simulink model "raibert_controller_running"  (R2018b)
settings: Solver=FixedStepDiscrete  StartTime=0.0  StopTime=inf  FixedStep=sample_time  RelTol=1e-3
InitFcn:
  | warning off all
undefined symbols (not defined in the file or in its folder): ctrl, Discrete, initial_dx_estimate, initial_dy_estimate, initial_dz_estimate, initial_z_estimate, sample_time, Time
libraries: simulink x27, ctrlSharedLib x7
(part 4 of 4)

== matlab function raibert_controller_running/Behavior/Primary-Secondary Routing Inputs ==
  data: right_is_primary input size=1; leg_angle_primary output size=2; leg_angle_right input size=2; leg_length_right input size=2; leg_width_right input size=2; leg_roll_right input size=2; back_load_right input size=2; back_motor_right input size=2; front_load_right input size=2; front_motor_right input size=2; lateral_right input size=2; axial_force_right input; grf_xz_right input; foot2com_x_right input; foot2com_z_right input; x_state_right input; leg_angle_left input size=2; leg_length_left input size=2; leg_width_left input size=2; leg_roll_left input size=2; back_load_left input size=2; back_motor_left input size=2; front_load_left input size=2; front_motor_left input size=2; lateral_left input size=2; leg_length_primary output size=2; leg_width_primary output size=2; leg_roll_primary output size=2; back_load_primary output size=2; back_motor_primary output size=2; front_load_primary output size=2; front_motor_primary output size=2; lateral_primary output size=2; axial_force_primary output; grf_xz_primary output; foot2com_x_primary output; foot2com_z_primary output; x_state_primary output; leg_angle_secondary output size=2; leg_length_secondary output size=2; leg_width_secondary output size=2; leg_roll_secondary output size=2; back_load_secondary output size=2; back_motor_secondary output size=2; front_load_secondary output size=2; front_motor_secondary output size=2; lateral_secondary output size=2; axial_force_left input; grf_xz_left input; foot2com_x_left input; foot2com_z_left input; axial_force_secondary output; grf_xz_secondary output; foot2com_x_secondary output; foot2com_z_secondary output; x_state_secondary output; x_state_left input
% Switch between "primary" and "secondary" leg variables
function [leg_angle_primary, ...
          leg_length_primary, ...
          leg_width_primary, ...
          leg_roll_primary, ...
          back_load_primary, ...
          back_motor_primary, ...
          front_load_primary, ...
          front_motor_primary, ...
          lateral_primary, ...
          axial_force_primary, ...
          grf_xz_primary, ...
          foot2com_x_primary, ...
          foot2com_z_primary, ...
          x_state_primary, ...
          leg_angle_secondary, ...
          leg_length_secondary, ...
          leg_width_secondary, ...
          leg_roll_secondary, ...
          back_load_secondary, ...
          back_motor_secondary, ...
          front_load_secondary, ...
          front_motor_secondary, ...
          lateral_secondary, ...
          axial_force_secondary, ...
          grf_xz_secondary, ...
          foot2com_x_secondary, ...
          foot2com_z_secondary, ...
          x_state_secondary] ...
          = SignalSwitch(...
          right_is_primary, ...
          leg_angle_right, ...
          leg_length_right, ...
          leg_width_right, ...
          leg_roll_right, ...
          back_load_right, ...
          back_motor_right, ...
          front_load_right, ...
          front_motor_right, ...
          lateral_right, ...
          axial_force_right, ...
          grf_xz_right, ...
          foot2com_x_right, ...
          foot2com_z_right, ...
          x_state_right, ...
          leg_angle_left, ...
          leg_length_left, ...
          leg_width_left, ...
          leg_roll_left, ...
          back_load_left, ...
          back_motor_left, ...
          front_load_left, ...
          front_motor_left, ...
          lateral_left, ...
          axial_force_left, ...
          grf_xz_left, ...
          foot2com_x_left, ...
          foot2com_z_left, ...
          x_state_left)

if right_is_primary % right leg is primary
  leg_angle_primary = leg_angle_right;
  leg_length_primary = leg_length_right;
  leg_width_primary = leg_width_right;
  leg_roll_primary = leg_roll_right;
  back_load_primary = back_load_right;
  back_motor_primary = back_motor_right;
  front_load_primary = front_load_right;
  front_motor_primary = front_motor_right;
  lateral_primary = lateral_right;
  axial_force_primary = axial_force_right;
  grf_xz_primary = grf_xz_right;
  foot2com_x_primary = foot2com_x_right;
  foot2com_z_primary = foot2com_z_right;
  x_state_primary = x_state_right;
  leg_angle_secondary = leg_angle_left;
  leg_length_secondary = leg_length_left;
  leg_width_secondary = leg_width_left;
  leg_roll_secondary = leg_roll_left;
  back_load_secondary = back_load_left;
  back_motor_secondary = back_motor_left;
  front_load_secondary = front_load_left;
  front_motor_secondary = front_motor_left;
  lateral_secondary = lateral_left;
  axial_force_secondary = axial_force_left;
  grf_xz_secondary = grf_xz_left;
  foot2com_x_secondary = foot2com_x_left;
  foot2com_z_secondary = foot2com_z_left;
  x_state_secondary = x_state_left;
else % left leg is primary
  leg_angle_primary = leg_angle_left;
  leg_length_primary = leg_length_left;
  leg_width_primary = leg_width_left;
  leg_roll_primary = leg_roll_left;
  back_load_primary = back_load_left;
  back_motor_primary = back_motor_left;
  front_load_primary = front_load_left;
  front_motor_primary = front_motor_left;
  lateral_primary = lateral_left;
  axial_force_primary = axial_force_left;
  grf_xz_primary = grf_xz_left;
  foot2com_x_primary = foot2com_x_left;
  foot2com_z_primary = foot2com_z_left;
  x_state_primary = x_state_left;
  leg_angle_secondary = leg_angle_right;
  leg_length_secondary = leg_length_right;
  leg_width_secondary = leg_width_right;
  leg_roll_secondary = leg_roll_right;
  back_load_secondary = back_load_right;
  back_motor_secondary = back_motor_right;
  front_load_secondary = front_load_right;
  front_motor_secondary = front_motor_right;
  lateral_secondary = lateral_right;
  axial_force_secondary = axial_force_right;
  grf_xz_secondary = grf_xz_right;
  foot2com_x_secondary = foot2com_x_right;
  foot2com_z_secondary = foot2com_z_right;
  x_state_secondary = x_state_right;
end

== matlab function raibert_controller_running/Behavior/Filtering/Kalman Filtering/Measurement Noise Covariance Matricies ==
  data: R_no_position output; R_transverse_right output; R_transverse_left output; vertical_GRF_L input; vertical_GRF_R input; sample_time parameter; ctrl parameter; R_vertical output
function [R_no_position, R_transverse_right, R_transverse_left, R_vertical] =...
         MeasurementNoiseCovariance(vertical_GRF_L, vertical_GRF_R, ...
         sample_time, ctrl)

    % filter states: [dx_w]; [dy_w]; [dz_w];
    % measurements:  [dx_w-dfL + dfL_hat; dx_w-dfR + dfR_hat]; 

    ratio_L = max(0, min(vertical_GRF_L/(ctrl.kalman_stance_slip_threshold*ctrl.m_total*ctrl.g),1)); % ratio is 0 if no load, 1 if at least equilibrium
    ratio_R = max(0, min(vertical_GRF_R/(ctrl.kalman_stance_slip_threshold*ctrl.m_total*ctrl.g),1));
    R_transverse_right = diag([ratio_R*ctrl.R_kalman_foot_stance + (1-ratio_R)*ctrl.R_kalman_foot_slip, ...
                               ctrl.R_kalman_accelerometer])/sample_time;
    R_transverse_left = diag([ratio_L*ctrl.R_kalman_foot_stance + (1-ratio_L)*ctrl.R_kalman_foot_slip, ...
                              ctrl.R_kalman_accelerometer])/sample_time;            
    R_vertical = diag([ratio_L*ctrl.R_kalman_foot_stance  + (1-ratio_L)*ctrl.R_kalman_foot_slip,...
                       ratio_R*ctrl.R_kalman_foot_stance  + (1-ratio_R)*ctrl.R_kalman_foot_slip,...
                       ctrl.R_kalman_accelerometer])/sample_time;
                   
    R_no_position = diag([ratio_L*ctrl.R_kalman_dfoot_stance + (1-ratio_L)*ctrl.R_kalman_dfoot_slip, ...
                          ratio_R*ctrl.R_kalman_dfoot_stance + (1-ratio_R)*ctrl.R_kalman_dfoot_slip, ...
                          ctrl.R_kalman_accelerometer])/sample_time;
end

== matlab function raibert_controller_running/Behavior/Convert to Body Frame IMU Accelerations ==
  data: accelerometer input; imu_accelerations output; ctrl parameter
function imu_accelerations = imu_to_body_frame(accelerometer, ctrl)
    z_up_rotation = [1, 0, 0; 0, 0, 1; 0, -1, 0];
    align_xy_rotation = [sqrt(2)/2, -sqrt(2)/2, 0; sqrt(2)/2, sqrt(2)/2, 0; 0, 0, 1];
    imu_accelerations = ctrl.g*z_up_rotation*align_xy_rotation*accelerometer;
end

== matlab function raibert_controller_running/Behavior/SEA Measurements/Leg Dynamics Left ==
  data: tau_back input; tau_front input; axial_force output; leg_width input; leg_length input; ortho_force output
function [axial_force, ortho_force] = fcn(tau_back, tau_front, leg_width, leg_length)

  % prevent divide by zero
  leg_width(1) = max(leg_width(1),eps);
  leg_length(1) = max(leg_length(1),eps);

  % forces and torques
  hip_torque = tau_front + tau_back;
  spread_torque = tau_front - tau_back;
  axial_force = zeros(2,1);
  axial_force(1) = spread_torque(1) / leg_width(1);
  ortho_force = zeros(2,1);
  ortho_force(1) = hip_torque(1) / leg_length(1);
  
  % time derivatives
  axial_force(2) = (leg_width(1)*spread_torque(2) - spread_torque(1)*leg_width(2)) / (leg_width(1)*leg_width(1));
  ortho_force(2) = (leg_length(1)*hip_torque(2) - hip_torque(1)*leg_length(2)) / (leg_length(1)*leg_length(1));
  
end

== matlab function raibert_controller_running/Behavior/Leg Plane GRF Right/World Frame React Forces ==
  data: F_horz output; leg_angle input; F_vert output; torso_pitch input; F_axial input; F_ortho input
function [F_horz, F_vert] = fcn(leg_angle, torso_pitch, F_axial, F_ortho)

  % define world frame leg angle
  gamma = leg_angle + torso_pitch;

  % compute forces
  F_vert = zeros(2,1);
  F_horz = zeros(2,1);
  F_vert(1) = -F_axial(1)*cos(gamma(1)) + F_ortho(1)*sin(gamma(1));
  F_horz(1) = -F_axial(1)*sin(gamma(1)) - F_ortho(1)*cos(gamma(1));
  
  % compute time derivatives
  F_vert(2) =  gamma(2)*(F_axial(1)*sin(gamma(1)) + F_ortho(1)*cos(gamma(1))) - F_axial(2)*cos(gamma(1)) + F_ortho(2)*sin(gamma(1));
  F_horz(2) =  gamma(2)*(-F_axial(1)*cos(gamma(1)) + F_ortho(1)*sin(gamma(1))) - F_axial(2)*sin(gamma(1)) - F_ortho(2)*cos(gamma(1));
  
end

== matlab function raibert_controller_running/Behavior/Leg Plane GRF Left/World Frame React Forces ==
  data: F_horz output; leg_angle input; F_vert output; torso_pitch input; F_axial input; F_ortho input
function [F_horz, F_vert] = fcn(leg_angle, torso_pitch, F_axial, F_ortho)

  % define world frame leg angle
  gamma = leg_angle + torso_pitch;

  % compute forces
  F_vert = zeros(2,1);
  F_horz = zeros(2,1);
  F_vert(1) = -F_axial(1)*cos(gamma(1)) + F_ortho(1)*sin(gamma(1));
  F_horz(1) = -F_axial(1)*sin(gamma(1)) - F_ortho(1)*cos(gamma(1));
  
  % compute time derivatives
  F_vert(2) =  gamma(2)*(F_axial(1)*sin(gamma(1)) + F_ortho(1)*cos(gamma(1))) - F_axial(2)*cos(gamma(1)) + F_ortho(2)*sin(gamma(1));
  F_horz(2) =  gamma(2)*(-F_axial(1)*cos(gamma(1)) + F_ortho(1)*sin(gamma(1))) - F_axial(2)*sin(gamma(1)) - F_ortho(2)*cos(gamma(1));
  
end

== matlab function raibert_controller_running/Behavior/Swing Leg Control Secondary/Virtual Leg to Four Bar ==
  data: l_leg input; dl_leg input; ddl_leg input; phi input; dphi input; ddphi input; back output; dback output; ddback output; front output; dfront output; ddfront output
function [back, dback, ddback, front, dfront, ddfront] = VirtualLegToFourBar(l_leg, dl_leg, ddl_leg, phi, dphi, ddphi)
    [back, dback, ddback, front, dfront, ddfront] = VirtualLegToFourBar(l_leg, dl_leg, ddl_leg, phi, dphi, ddphi);
end

== matlab function raibert_controller_running/Behavior/Raibert Controller/Plan Swing Leg Trajectories/Plan Swing Trajectories ==
  data: enable input; replan input; t_plan input; phase input; com_x_velocity input; z_state input; foot2com_x_primary input; foot2com_z_primary input; foot2com_x_secondary input; foot2com_z_secondary input; right_is_primary input; neutral_point input; k_placement input; desired_x_primary output; desired_y_primary output; desired_z_primary output; desired_x_secondary output; desired_y_secondary output; desired_z_secondary output; ctrl parameter
% Plan Foot2CoM trajectories in XYZ space for the swing phase
function [desired_x_primary, desired_y_primary, desired_z_primary, ...
          desired_x_secondary, desired_y_secondary, desired_z_secondary] = ...
          PlanFeet(enable, replan, ...
                    t_plan, phase, com_x_velocity, z_state, ...
                    foot2com_x_primary, foot2com_z_primary, ...
                    foot2com_x_secondary, foot2com_z_secondary, ...
                    right_is_primary, neutral_point, k_placement, ...
                    ctrl)
                  
  % not applicable in double support (return zero)
%     if phase == 2
%       desired_x_primary = [0 0 0]';
%       desired_y_primary = [0 0 0]';
%       desired_z_primary = [0 0 0]';
%       desired_x_secondary = [0 0 0]';
%       desired_y_secondary = [0 0 0]';
%       desired_z_secondary = [0 0 0]';
%       return;
%     end

  % persistent variables to store swing foot plan(s) as splines in (X,Z) space
  persistent ax bx cx dx az1 bz1 cz1 dz1 az2 bz2 cz2 dz2 ...
             t_final x0_pos x0_vel xf_vel

  % plan swing feet
  if isempty(ax) || replan
    % convert (leg_length, leg_angle) space to (X,Z) space
%     x_target = neutral_point + k_placement * (ctrl.com_x_vel_desired - com_x_velocity);
    z_target = ctrl.z_swing_target;
    if phase == 0 % Flight (plan primary and secondary legs)
      % calculate swing time in flight
      t_final = (z_state(2) + sqrt(max(z_state(2)^2 - 2*ctrl.g*(z_target-z_state(1)),0)))/ctrl.g;
      t_min = abs(z_target - foot2com_z_primary(1)) / ctrl.max_vert_swing_speed;
      t_final = max(t_final, t_min); % lower bound swing time
      % primary x trajectory during flight
      x_target = -0.5*t_final*com_x_velocity + k_placement * (ctrl.com_x_vel_desired - com_x_velocity);
      x0_pos = foot2com_x_primary(1); 
      x0_vel = foot2com_x_primary(2);
      xf_pos = x_target;
      xf_vel = com_x_velocity; % match horizontal ground speed in flight
      [ ax, bx, cx, dx ] = ThirdOrderTrajectory( x0_pos, x0_vel, xf_pos, xf_vel, t_final );
      % primary z trajectory during flight
      z0_pos = foot2com_z_primary(1);
      z0_vel = foot2com_z_primary(2);
      zf_pos = z_target;
      zf_vel = 0;
      [ az1, bz1, cz1, dz1 ] = ThirdOrderTrajectory( z0_pos, z0_vel, zf_pos, zf_vel, t_final );
      az2 = 0; bz2 = 0; cz2 = 0; dz2 = 0;
    else % phase == 1 % single support
      % plan until initial double support
      t_final = ctrl.reactive_swing_time;
      % secondary x trajectory
      x_target = -0.5*t_final*com_x_velocity + k_placement * (ctrl.com_x_vel_desired - com_x_velocity);
      x0_pos = foot2com_x_secondary(1); 
      x0_vel = foot2com_x_secondary(2);
      xf_pos = x_target;
      xf_vel = 0;
      [ ax, bx, cx, dx ] = ThirdOrderTrajectory( x0_pos, x0_vel, xf_pos, xf_vel, t_final );
      % secondary z trajectory
      z0_pos = foot2com_z_secondary(1);
      z0_vel = foot2com_z_secondary(2);
      zmid_pos = z_target - ctrl.max_z_retract;
      zmid_vel = 0;
      [ az1, bz1, cz1, dz1 ] = ThirdOrderTrajectory( z0_pos, z0_vel, zmid_pos, zmid_vel, 0.5*t_final );
      zf_vel = 0;
      [ az2, bz2, cz2, dz2 ] = ThirdOrderTrajectory( zmid_pos, zmid_vel, z_target, zf_vel, 0.5*t_final );
    end
  end
  
  % y target varies from left to right side of robot
  if right_is_primary
    y_swing_target_1 = ctrl.y_swing_target_right;
    y_swing_target_2 = ctrl.y_swing_target_left;
  else
    y_swing_target_1 = ctrl.y_swing_target_left;
    y_swing_target_2 = ctrl.y_swing_target_right;
  end
  
  % compute reference from polynomials if enabled
  if enable
    % bound the time
    trajectory_valid = t_plan <= t_final;
    t_plan = min(max(t_plan,0),t_final);
    % replan using feedback policy
%     xf_pos = neutral_point + k_placement * (ctrl.com_x_vel_desired - com_x_velocity);
    xf_pos = -0.5 * t_final * com_x_velocity + k_placement * (ctrl.com_x_vel_desired - com_x_velocity);
    xf_pos = min(max(xf_pos, -0.5), 0.5);
    [ ax, bx, cx, dx ] = ThirdOrderTrajectory( x0_pos, x0_vel, xf_pos, xf_vel, t_final );
    % compute x reference
    x_pos = ax*t_plan^3 + bx*t_plan^2 + cx*t_plan + dx;
    x_vel = trajectory_valid*(3*ax*t_plan^2 + 2*bx*t_plan + cx);
    x_acc = trajectory_valid*(6*ax*t_plan + 2*bx);
    % compute other references in flight
    if phase == 0
      % primary z
      z_pos_1 = az1*t_plan^3 + bz1*t_plan^2 + cz1*t_plan + dz1;
      z_vel_1 = trajectory_valid*(3*az1*t_plan^2 + 2*bz1*t_plan + cz1);
      z_acc_1 = trajectory_valid*(6*az1*t_plan + 2*bz1);
      % secondary x (reflect over x = 0)
      x_pos_2 = -x_pos;
      x_vel_2 = -x_vel;
      x_acc_2 = -x_acc;
      % secondary z
      z_pos_2 = z_pos_1 - ctrl.z_retract_flight;
      z_vel_2 = z_vel_1;
      z_acc_2 = z_acc_1;
      % assign references to outputs
      desired_x_primary = [x_pos; x_vel; x_acc];
      desired_y_primary = [y_swing_target_1; 0; 0];
      desired_z_primary = [z_pos_1; z_vel_1; z_acc_1];
      desired_x_secondary = [x_pos_2; x_vel_2; x_acc_2];
      desired_y_secondary = [y_swing_target_2; 0; 0];
      desired_z_secondary = [z_pos_2; z_vel_2; z_acc_2];
    else % compute z references in single support
      if t_plan < 0.5*t_final % retraction
        z_pos = az1*t_plan^3 + bz1*t_plan^2 + cz1*t_plan + dz1;
        z_vel = trajectory_valid*(3*az1*t_plan^2 + 2*bz1*t_plan + cz1);
        z_acc = trajectory_valid*(6*az1*t_plan + 2*bz1); 
      else % extension
        t_plan = t_plan - 0.5*t_final;
        z_pos = az2*t_plan^3 + bz2*t_plan^2 + cz2*t_plan + dz2;
        z_vel = trajectory_valid*(3*az2*t_plan^2 + 2*bz2*t_plan + cz2);
        z_acc = trajectory_valid*(6*az2*t_plan + 2*bz2);
      end
      % assign references to outputs
      desired_x_primary = [0; 0; 0];
      desired_y_primary = [0; 0; 0];
      desired_z_primary = [0; 0; 0];
      desired_x_secondary = [x_pos; x_vel; x_acc];
      desired_y_secondary = [y_swing_target_2; 0; 0];
      desired_z_secondary = [z_pos; z_vel; z_acc];
    end

  else % default primary target if disabled
    desired_x_primary = [ctrl.initial_x_pos_swing 0 0]';
    desired_y_primary = [y_swing_target_1 0 0]';
    desired_z_primary = [ctrl.initial_z_pos_swing 0 0]';
    desired_x_secondary = -desired_x_primary;
    desired_y_secondary = [y_swing_target_2 0 0]';
    desired_z_secondary = desired_z_primary - ctrl.z_retract_flight;
  end
  
end

== matlab function raibert_controller_running/Behavior/CoM Kinematics/PositionUsingRobotGeometry ==
  data: com_left_yawed output; dcom_left_yawed output; com_right_yawed output; dcom_right_yawed output; roll input; pitch input; yaw input; left_leg_sagittal_angle input; left_leg_lateral_angle input; left_leg_length input; right_leg_sagittal_angle input; right_leg_lateral_angle input; right_leg_length input; com_left_global output; dcom_left_global output; ctrl parameter; com_right_global output; dcom_right_global output; com_pelvis_body output; dcom_pelvis_body output
% Returns CoM relative to primary foot
function [com_left_yawed, dcom_left_yawed, ...
          com_right_yawed, dcom_right_yawed, ...
          com_left_global, dcom_left_global, ...
          com_right_global, dcom_right_global, ...
          com_pelvis_body, dcom_pelvis_body] = ...
         ComPositionUsingRobotGeometry(roll, pitch, yaw, ...
                           left_leg_sagittal_angle, left_leg_lateral_angle, left_leg_length, ...
                           right_leg_sagittal_angle, right_leg_lateral_angle, right_leg_length, ...
                           ctrl)
                    
  q =  [roll(1), pitch(1), yaw(1), ...
        left_leg_sagittal_angle(1), left_leg_lateral_angle(1), left_leg_length(1), ...
        right_leg_sagittal_angle(1), right_leg_lateral_angle(1), right_leg_length(1)];
  dq = [roll(2), pitch(2), yaw(2), ...
        left_leg_sagittal_angle(2), left_leg_lateral_angle(2), left_leg_length(2), ...
        right_leg_sagittal_angle(2), right_leg_lateral_angle(2), right_leg_length(2)];

  [ com_pelvis, dcom_pelvis, ...
    com_left, dcom_left, ...
    com_right, dcom_right ] = ...
  ComCalculationFromRobot( q, dq, ctrl.m_torso, ctrl.m_leg_motor, ctrl.m_leg, ctrl.com_torso, ...
                           ctrl.com_leg_motor, ctrl.lateral_offset );
  
  % left foot measurements
  com_left_yawed = com_left(4:6);
  com_left_global = com_left(7:9);
  dcom_left_yawed = dcom_left(4:6);
  dcom_left_global = dcom_left(7:9);
  
  % right foot measurements
  com_right_yawed = com_right(4:6);
  com_right_global = com_right(7:9);
  dcom_right_yawed = dcom_right(4:6);
  dcom_right_global = dcom_right(7:9);
  
  % pelvis measurement
  com_pelvis_body = com_pelvis(1:3);
  dcom_pelvis_body = dcom_pelvis(1:3);
  
end

== matlab function raibert_controller_running/Behavior/Primary-Secondary Routing Outputs ==
  data: right_is_primary input size=1; joint_torque_primary input size=2; motor_velocity_primary input size=2; lateral_torque_primary input size=1; joint_torque_secondary input size=2; motor_velocity_secondary input size=2; lateral_torque_secondary input size=1; joint_torque_right output size=2; motor_velocity_right output size=2; lateral_torque_right output size=1; joint_torque_left output size=2; motor_velocity_left output size=2; lateral_torque_left output size=1
% Switch between "primary" and "secondary" leg variables
function [joint_torque_right, ...
          motor_velocity_right, ...
          lateral_torque_right, ...
          joint_torque_left, ...
          motor_velocity_left, ...
          lateral_torque_left] ...
          = SignalSwitch(...
          right_is_primary, ...
          joint_torque_primary, ...
          motor_velocity_primary, ...
          lateral_torque_primary, ...
          joint_torque_secondary, ...
          motor_velocity_secondary, ...
          lateral_torque_secondary)

if right_is_primary % right leg is primary
  joint_torque_right = joint_torque_primary;
  motor_velocity_right = motor_velocity_primary;
  lateral_torque_right = lateral_torque_primary;
  joint_torque_left = joint_torque_secondary;
  motor_velocity_left = motor_velocity_secondary;
  lateral_torque_left = lateral_torque_secondary;
else % left leg is primary
  joint_torque_right = joint_torque_secondary;
  motor_velocity_right = motor_velocity_secondary;
  lateral_torque_right = lateral_torque_secondary;
  joint_torque_left = joint_torque_primary;
  motor_velocity_left = motor_velocity_primary;
  lateral_torque_left = lateral_torque_primary;
end

== matlab function raibert_controller_running/Behavior/Swing Leg Control Primary/Avoid Hitting Mechanical Limits ==
  data: back_cmd output double; front_cmd output double; dback_cmd output double; dfront_cmd output double; ddback_cmd output double; ddfront_cmd output double; back_desired input; dback_desired input; ddback_desired input; front_desired input; dfront_desired input; ddfront_desired input; ctrl parameter
%% Avoid fourbar limits by saturating the commands and ensuring we don't command velocities or 
% accelerations that would push us into the limits when nearby
function [back_cmd, front_cmd, dback_cmd, dfront_cmd, ddback_cmd, ddfront_cmd] ...
    = AvoidFourbarLimits(back_desired,dback_desired, ddback_desired, ...
          front_desired, dfront_desired, ddfront_desired, ...
          ctrl)
    [back_cmd, front_cmd, dback_cmd, dfront_cmd, ddback_cmd, ddfront_cmd] = ...
      AvoidFourbarLimits(back_desired, dback_desired, ddback_desired, ...
                         front_desired, dfront_desired, ddfront_desired, ...
                         ctrl.min_front_bar_angle, ctrl.max_front_bar_angle, ...
                         ctrl.min_back_bar_angle, ctrl.max_back_bar_angle);
end

== matlab function raibert_controller_running/Behavior/Swing Leg Control Secondary/Avoid Virtual Leg Length Limits ==
  data: l_leg_desired input; dl_leg_desired input; ddl_leg_desired input; l_leg_cmd output double; dl_leg_cmd output double; ddl_leg_cmd output double; ctrl parameter
%% Avoid virtual leg length limits by ensuring we don't command position/velocities/accelerations that would hit them.
function [l_leg_cmd, dl_leg_cmd, ddl_leg_cmd] = ...
  AvoidVirtualLengthLimits(l_leg_desired, dl_leg_desired, ddl_leg_desired, ctrl)
    [l_leg_cmd, dl_leg_cmd, ddl_leg_cmd] = ...
      AvoidVirtualLengthLimits(l_leg_desired, dl_leg_desired, ddl_leg_desired, ...
                               ctrl.min_leg_length, ctrl.max_leg_length);
end

== matlab function raibert_controller_running/Behavior/Swing Leg Control Primary/Avoid Virtual Leg Length Limits ==
  data: l_leg_desired input; dl_leg_desired input; ddl_leg_desired input; l_leg_cmd output double; dl_leg_cmd output double; ddl_leg_cmd output double; ctrl parameter
%% Avoid virtual leg length limits by ensuring we don't command position/velocities/accelerations that would hit them.
function [l_leg_cmd, dl_leg_cmd, ddl_leg_cmd] = ...
  AvoidVirtualLengthLimits(l_leg_desired, dl_leg_desired, ddl_leg_desired, ctrl)
    [l_leg_cmd, dl_leg_cmd, ddl_leg_cmd] = ...
      AvoidVirtualLengthLimits(l_leg_desired, dl_leg_desired, ddl_leg_desired, ...
                               ctrl.min_leg_length, ctrl.max_leg_length);
end

== matlab function raibert_controller_running/Behavior/Swing Leg Control Primary/Convert CoM (X,Y,Z) to  (Leg Angles, Leg Length) ==
  data: desired_leg_length output; X_star input; Y_star input; Z_star input; right_left input; pelvis2com_pos input; desired_alpha output; desired_beta output; pelvis2com_vel input; roll input; pitch input; sagittal_angle input; lateral_angle input; leg_length input; ctrl parameter
%% Convert Foot2CoM vector from (X, Y, Z) to (leg length, leg angle) space
function [ desired_leg_length, desired_alpha, desired_beta ]  =  ...
          ConvertToJointAnglesAndLegLength(X_star, Y_star, Z_star, right_left,...
                           pelvis2com_pos, pelvis2com_vel, ...
                           roll, pitch, sagittal_angle, lateral_angle, leg_length,...
                           ctrl) 

    q = [roll(1), pitch(1), sagittal_angle(1), lateral_angle(1), leg_length(1)];
    dq = [roll(2), pitch(2), sagittal_angle(2), lateral_angle(2), leg_length(2)];
    [desired_alpha, desired_beta, desired_leg_length] = ...
      ConvertComPositionToLegAnglesAndLegLength(X_star, Y_star, Z_star, right_left, ...
                                                pelvis2com_pos, pelvis2com_vel, ...
                                                q, dq, ctrl.lateral_offset);
    desired_beta = saturate(desired_beta, ctrl.min_lateral_beta, ctrl.max_lateral_beta);
end

function [desired_saturated] = saturate(desired, min_lateral_beta, max_lateral_beta)
    desired_saturated = desired;
    if desired(1) < min_lateral_beta
        desired_saturated = [min_lateral_beta; 0; 0];
    elseif desired(1) > max_lateral_beta
        desired_saturated = [max_lateral_beta; 0; 0];    
    end
end

== matlab function raibert_controller_running/Behavior/Swing Leg Control Primary/Virtual Leg to Four Bar ==
  data: l_leg input; dl_leg input; ddl_leg input; phi input; dphi input; ddphi input; back output; dback output; ddback output; front output; dfront output; ddfront output
function [back, dback, ddback, front, dfront, ddfront] = VirtualLegToFourBar(l_leg, dl_leg, ddl_leg, phi, dphi, ddphi)
    [back, dback, ddback, front, dfront, ddfront] = VirtualLegToFourBar(l_leg, dl_leg, ddl_leg, phi, dphi, ddphi);
end

== matlab function raibert_controller_running/Behavior/Tranform Sensor Measurements to CoM Acceleration Measurement/Compute CoM Translational Acceleration ==
  data: com_acceleration_yawed output; torso_com_acceleration_yawed output; pelvis_acceleration_yawed output; torso_angular_accelerations input; imu_translational_accelerations_body input; torso_roll input; torso_pitch input; hip_roll_accelerations input; right_hip_roll input; left_hip_roll input; ctrl parameter; right_hip_acceleration_yawed output; left_hip_acceleration_yawed output
%% Compute translational acceleration of the CoM from torso accelerometer and joint encoders
% (IMU uses non-rotating measurement frame)
function [com_acceleration_yawed, torso_com_acceleration_yawed, pelvis_acceleration_yawed, ...
          right_hip_acceleration_yawed, left_hip_acceleration_yawed] ...
          = compute_com_acceleration( torso_angular_accelerations, ...
                                      imu_translational_accelerations_body, ...
                                      torso_roll, torso_pitch, ...
                                      hip_roll_accelerations, right_hip_roll, left_hip_roll, ...
                                      ctrl)
    
    % Body frame to Yawed frame rotation matrices
    R_body_to_yawed = R_pitch(torso_pitch(1))*R_roll(torso_roll(1));
    dR_body_to_yawed = dR_pitch(torso_pitch(1),torso_pitch(2))*R_roll(torso_roll(1)) + R_pitch(torso_pitch(1))*dR_roll(torso_roll(1),torso_roll(2));
    ddR_body_to_yawed = ddR_pitch(torso_pitch(1),torso_pitch(2),torso_angular_accelerations(2))*R_roll(torso_roll(1)) ...
                        + R_pitch(torso_pitch(1))*ddR_roll(torso_roll(1),torso_roll(2),torso_angular_accelerations(1)) ... 
                        + 2*dR_pitch(torso_pitch(1),torso_pitch(2))*dR_roll(torso_roll(1),torso_roll(2));
    % Compute translational acceleration of torso COM in yawed frame
    imu_to_torso_com_acceleration_yawed = ddR_body_to_yawed*(ctrl.com_torso - ctrl.pelvis_to_imu)';
    imu_acceleration_yawed = R_body_to_yawed*imu_translational_accelerations_body;
    torso_com_acceleration_yawed = imu_acceleration_yawed + imu_to_torso_com_acceleration_yawed;
    % Compute accelerations of hip COMs
    R_right_hip_to_body =     R_roll(-pi/2+right_hip_roll(1));
    dR_right_hip_to_body =   dR_roll(-pi/2+right_hip_roll(1), right_hip_roll(2));
    ddR_right_hip_to_body = ddR_roll(-pi/2+right_hip_roll(1), right_hip_roll(2), hip_roll_accelerations(1));
    R_left_hip_to_body =     R_roll(pi/2-left_hip_roll(1));
    dR_left_hip_to_body =   dR_roll(pi/2-left_hip_roll(1), -left_hip_roll(2));
    ddR_left_hip_to_body = ddR_roll(pi/2-left_hip_roll(1), -left_hip_roll(2), -hip_roll_accelerations(2));
    imu_to_pelvis_com_acceleration_yawed = ddR_body_to_yawed*(-ctrl.pelvis_to_imu)';  
    pelvis_acceleration_yawed = imu_acceleration_yawed + imu_to_pelvis_com_acceleration_yawed;
    left_hip_acceleration_yawed = pelvis_acceleration_yawed + (ddR_body_to_yawed*R_left_hip_to_body + 2*dR_body_to_yawed*dR_left_hip_to_body + R_body_to_yawed*ddR_left_hip_to_body)*ctrl.com_leg_motor';
    right_hip_acceleration_yawed = pelvis_acceleration_yawed + (ddR_body_to_yawed*R_right_hip_to_body + 2*dR_body_to_yawed*dR_right_hip_to_body + R_body_to_yawed*ddR_right_hip_to_body)*(ctrl.com_leg_motor.*[1,-1,1])';
    % Compute total system COM acceleration
    m_hip = ctrl.m_leg+ctrl.m_leg_motor;
    m_total = 2*m_hip + ctrl.m_torso;
    com_acceleration_yawed = (ctrl.m_torso*torso_com_acceleration_yawed + m_hip*(left_hip_acceleration_yawed + right_hip_acceleration_yawed))/m_total;
    
end

function R_yp = R_pitch(theta) % map from pitched to yawed
  R_yp = [cos(theta), 0, sin(theta); ...
          0, 1, 0; ...
          -sin(theta), 0, cos(theta)];
end
function dR_yp = dR_pitch(theta,dtheta)
  dR_yp = dtheta*[-sin(theta), 0, cos(theta); ...
                  0, 0, 0; ... 
                  -cos(theta), 0, -sin(theta)];
end
function ddR_yp = ddR_pitch(theta,dtheta,ddtheta)
  ddR_yp = ddtheta*[-sin(theta), 0, cos(theta); ...
                    0, 0, 0; ... 
                    -cos(theta), 0, -sin(theta)] ...
           + dtheta^2*[-cos(theta), 0, -sin(theta); ...
                     0, 0, 0; ...
                     sin(theta), 0, -cos(theta)];
end
function R_pr = R_roll(phi) % map from rolled to pitched
  R_pr = [1, 0, 0; ...
          0, cos(phi), -sin(phi); ...
          0, sin(phi), cos(phi)]; 
end
function dR_pr = dR_roll(phi,dphi)
  dR_pr = dphi*[0, 0, 0; ...
                0, -sin(phi), -cos(phi); ...
                0, cos(phi), -sin(phi)];
end
function ddR_pr = ddR_roll(phi, dphi, ddphi)
  ddR_pr = ddphi*[0, 0, 0; ...
                  0, -sin(phi), -cos(phi); ...
                  0, cos(phi), -sin(phi)] ...
           + dphi^2*[0, 0, 0; ...
                   0, -cos(phi), sin(phi);...
                   0, -sin(phi), -cos(phi)];
end
function R_gy = R_yaw(psi) % map yawed frame to global
  R_gy = [cos(psi), -sin(psi), 0; sin(psi), cos(psi), 0; 0 0 1]; 
end
function dR_gy = dR_yaw(psi,dpsi)
  dR_gy = dpsi*[-sin(psi), -cos(psi), 0; cos(psi), -sin(psi), 0; 0 0 0];
end
function ddR_gy = ddR_yaw(psi,dpsi,ddpsi)
  ddR_gy = ddpsi*[-sin(psi), -cos(psi), 0; cos(psi), -sin(psi), 0; 0 0 0] ...
           + dpsi^2*[-cos(psi), sin(psi), 0; -sin(psi), -cos(psi), 0; 0 0 0];
end
